simulink model "actuator_sensor"  (R2017a)
settings: Solver=ode45  StartTime=0.0  StopTime=150  FixedStep=1e-4  RelTol=1e-6  EnableMultiTasking=on
values from neighbouring files (symbols this model uses):
  A = [3.7451e-15 7.6548e-6 0 0;-4.0887e-6 -6.5527e-2 0 0;     2.3773e-6 5.9026e-4 -0.1426 0;-8.1593e-14 -5.5355e-2 18.216 0.08333];eig(A)    [boiler.m]    (also in boiler2.m = [3.7451e-15 7.6548e-6 0 0;-4.0887e-6 -6.5527e-2 0 0;     2.3)
  A0 = [zeros(3,2);A0]    [boiler2.m]
  A_m = [-0.01 0 0;0 -0.02 0;0 0 -0.03]    [boiler.m]    (also in boiler2.m)
  Ab = [A zeros(n,psi_s);Omega*C_f -Omega]    [boiler2.m]
  alpha_0 = 8.0314    [boiler.m]    (also in boiler2.m)
  alpha_1 = 1.4713    [boiler.m]    (also in boiler2.m)
  B = [0.0015 -0.0015 -6.9678e-12;-5.9548e-5 -9.0316e-5 5.9647e-11;     3.4622e-5 5.2512e-5 3.2492e-11;-0.0167 0.0239 -1.0733e-9]    [boiler.m]    (also in boiler2.m)
  B_m = [1 0 0 ; 0 1 0 ; 0 0 1]    [boiler.m]    (also in boiler2.m)
  Bb = [B;zeros(psi_s,m)]    [boiler2.m]
  Bound = 1e-3    (= 0.001)    [boiler.m]    (also in boiler2.m)
  C = [0.05 -0.0484 6.7129 0.05;0 1 0 0]    [boiler.m]    (also in boiler2.m)
  C_m = [0 1 0;1 0 0]    [boiler.m]    (also in boiler2.m)
  Cb = [C_h zeros(p-psi_s,psi_s);zeros(psi_s,n) eye(psi_s)]    [boiler2.m]
  D = [0 0 0 ; 0 0 0]    [boiler.m]    (also in boiler2.m = [0 0 0 20]')
  Db_p = T*Db    [boiler2.m]
  E = dB    [boiler2.m]
  f_a = 10    [boiler2.m]
  f_s = 0.1    [boiler2.m]
  FTC_factor = 1    [boiler2.m]
  G = [0.968,-114.258,-1;1,0,0;0,1,0;0,0,1]    [boiler.m]    (also in boiler2.m)
  gamma = 0.0013    [boiler.m]    (also in boiler2.m)
  Gamma = 1*diag([1,1,1])    [boiler.m]    (also in boiler2.m)
  H = [-0.00264411452837401,0.276368234354978,0.00485669922298695;-0.00212093673792562,0.126828183853013,0.00297639139790861;-11263.6759461726,221638.898137783,1282.33499200163]    [boiler.m]    (also in boiler2.m)
  k = norm(D2)*pa + eta1    [boiler2.m]
  K_D = [0.0691 0 0 0.0691;0 0.0691 0 0;0 0 0.0691 0]    [boiler.m]    (also in boiler2.m)
  K_I = 2*[eye(3),[1;0;0]]    [boiler.m]    (also in boiler2.m)
  K_P = .1*[eye(3),[1;0;0]]    [boiler.m]    (also in boiler2.m)
  K_S = 0.01*eye(3)    [boiler.m]    (also in boiler2.m)
  M = [0.322180266848393,-23.9048793908242,-0.198387888997022;0.273413353570640,-16.9472760226837,-0.136907357417107;1077571.96327408,-5503793.87571974,-55561.6496148715]    [boiler.m]    (also in boiler2.m)
  N = [0 1]'    [boiler2.m]
  Omega = 10    [boiler2.m]
  P0 = eye(p)    [boiler2.m]
  sai = 1e-3    (= 0.001)    [boiler2.m]
  T = [[eye(3) zeros(3,2)];Cb]    [boiler2.m]
  um_factor = 1    [boiler.m]    (also in boiler2.m = 0)
settings Model: Creator=Mohmmad Mousavi  LastModifiedBy=Mohmmad Mousavi
settings DataIOCC: LimitDataPoints=on  SaveFormat=Array
settings OptimizationCC: LifeSpan=inf
settings DebuggingCC: SFUnexpectedBacktrackingDiag=warning  SFNoUnconditionalDefaultTransitionDiag=warning  SFExecutionAtInitializationDiag=none
settings HardwareCC: ProdBitPerPointer=32  ProdBitPerSizeT=32  ProdBitPerPtrDiffT=32  ProdLargestAtomicFloat=None  ProdIntDivRoundTo=Undefined  ProdEndianess=Unspecified  ProdWordSize=32  ProdHWDeviceType=32-bit Generic
settings ModelReferenceCC: PropagateSignalLabelsOutOfModel=off
settings GRTTargetCC: TargetLangStandard=C89/C90 (ANSI)  GeneratePreprocessorConditionals=Disable all
settings ConfigComp: CovMetricSettings=dw  CovHtmlReporting=on  CovSaveCumulativeToWorkspaceVar=on  CovSaveSingleToWorkspaceVar=on  CovExternalEMLEnable=off

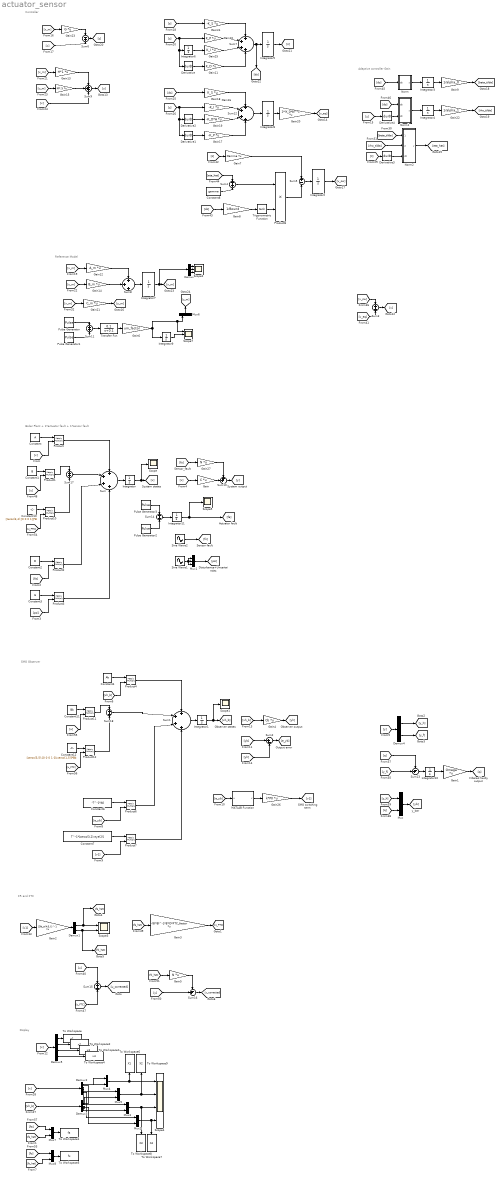
== system actuator_sensor ==
  note: FR and FTC
  note: Display
  note: Boiler Plant + 1*actuator fault + 1*sensor fault
  note: SMO Observer
  note: Controller
  note: Adaptive controller Gain
  note: Reference Model
  Constant : Constant  Value=A
  Constant1 : Constant  Value=B
  Constant10 : Constant  Value=[zeros(3,4);[0 0 0 1]]*B
  Constant11 : Constant  Value=Bb
  Constant12 : Constant  Value=[zeros(3,5);[0 0 0 1 0];zeros(1,5)]*Bb
  Constant2 : Constant  Value=D
  Constant3 : Constant  Value=E
  Constant4 : Constant  Value=Ab
  Constant6 : Constant  Value=-T^-1*A0
  Constant7 : Constant  Value=T^-1*[zeros(3,2);eye(2)]
  Constant8 : Constant  Value=gamma
  Demux : Demux  Outputs=3
  Demux1 : Demux  Outputs=2
  Demux2 : Demux  Outputs=n
  Demux3 : Demux  Outputs=5
  Demux4 : Demux  Outputs=2
  Demux5 : Demux  Outputs=n
  Derivative{,1..4} (5 alike) : Derivative
  Gain : Gain  Gain=C  Multiplication=Matrix(K*u)
  Gain1 : Gain  Gain=Omega  Multiplication=Matrix(K*u)
  Gain10 : Gain  Gain=K_P  Multiplication=Matrix(K*u)
  Gain11 : Gain  Gain=K_D  Multiplication=Matrix(K*u)
  Gain12 : Gain  Gain=A_m  Multiplication=Matrix(K*u)
  Gain13 : Gain  Gain=H*1  Multiplication=Matrix(K*u)
  Gain14 : Gain  Gain=B_m  Multiplication=Matrix(K*u)
  Gain15 : Gain  Gain=M*.5  Multiplication=Matrix(K*u)
  Gain16 : Gain  Gain=-K_I  Multiplication=Matrix(K*u)
  Gain17 : Gain  Gain=-K_P  Multiplication=Matrix(K*u)
  Gain18 : Gain  Gain=K_S  Multiplication=Matrix(K*u)
  Gain19 : Gain  Gain=-K_D*A  Multiplication=Matrix(K*u)
  Gain2 : Gain  Gain=[Db_p(4:5,:)]^-1  Multiplication=Matrix(K*u)
  Gain20 : Gain  Gain=2*(K_D*B)^-1  Multiplication=Matrix(K*u)
  Gain21 : Gain  Gain=C_m  Multiplication=Matrix(K*u)
  Gain22 : Gain  Gain=1/alpha_1
  Gain23 : Gain  Gain=G  Multiplication=Matrix(K*u)
  Gain24 : Gain  Gain=-K_S  Multiplication=Matrix(K*u)
  Gain25 : Gain  Gain=K_I  Multiplication=Matrix(K*u)
  Gain26 : Gain  Gain=k*P0  Multiplication=Matrix(K*u)
  Gain27 : Gain  Gain=N  Multiplication=Matrix(K*u)
  Gain3 : Gain  Gain=-(B'*B)^-1*B'*D*FTC_factor  Multiplication=Matrix(K*u)
  Gain4 : Gain  Gain=Cb  Multiplication=Matrix(K*u)
  Gain5 : Gain  Gain=N  Multiplication=Matrix(K*u)
  Gain6 : Gain  Gain=um_factor
  Gain7 : Gain  Gain=Gamma  Multiplication=Matrix(K*u)
  Gain8 : Gain  Gain=1/Bound
  Gain9 : Gain  Gain=1/alpha_0
  Integrator : Integrator  InitialCondition=[25 30 9 -950]*0.5
  Integrator1 : Integrator  InitialCondition=[25 30*.5 9*0.5 -950 0]*0.5
  Integrator{3..6,8,10..11} (7 alike) : Integrator
  Integrator2 : Integrator  InitialCondition=zeros(3,1)
  Integrator7 : Integrator  InitialCondition=[ 60 9 0.05]
  Integrator9 : Integrator  InitialCondition=35
  MATLAB Function : MATLAB Function  TreatAsAtomicUnit=on
  Mux{,2..5,7..8} (7 alike) : Mux  Inputs=2
  Mux1 : Mux  Inputs=3
  Mux6 : Mux  Inputs=3
  Norm : MATLAB Function  TreatAsAtomicUnit=on
  Norm1 : MATLAB Function  TreatAsAtomicUnit=on
  Norm2 : MATLAB Function  TreatAsAtomicUnit=on
  Product{,1..4,6..7,10..12} (10 alike) : Product  Multiplication=Matrix(*)
  Product8 : Product
  Pulse Generator : DiscretePulseGenerator  PulseType=Time based  Amplitude=1.9  Period=100  PulseWidth=50
  Pulse Generator1 : DiscretePulseGenerator  PulseType=Time based  Amplitude=-.5  Period=100  PulseWidth=50  PhaseDelay=50
  Pulse Generator2 : DiscretePulseGenerator  PulseType=Time based  Amplitude=-f_a/5  Period=10  PulseWidth=50  PhaseDelay=5
  Pulse Generator3 : DiscretePulseGenerator  PulseType=Time based  Amplitude=f_a/5  Period=10  PulseWidth=50
  Scope : Scope
  Scope1 : Scope
  Scope2 : Scope  NumInputPorts=3
  Scope3 : Scope  NumInputPorts=2
  Scope4 : Scope  NumInputPorts=4
  Scope5 : Scope
  Scope7 : Scope  NumInputPorts=3
  Sine Wave1 : Sin  Amplitude=sai  SampleTime=0
  Sine Wave2 : Sin  Amplitude=f_s  SampleTime=0
  Sum{,1,7,12} (4 alike) : Sum  Inputs=++++
  Sum10 : Sum  Inputs=++|
  Sum{3..4,11,14..15,17..18} (7 alike) : Sum
  Sum13 : Sum  Inputs=-+|
  Sum16 : Sum  Inputs=-+|
  Sum2 : Sum  Inputs=|+-
  Sum5 : Sum  Inputs=+-
  Sum6 : Sum  Inputs=-+
  Sum8 : Sum  Inputs=+++
  Sum9 : Sum  Inputs=+++
  To Workspace : ToWorkspace  VariableName=x1  SaveFormat=Timeseries  SampleTime=-1
  To Workspace1 : ToWorkspace  VariableName=fa  SaveFormat=Timeseries  SampleTime=-1
  To Workspace2 : ToWorkspace  VariableName=x2  SaveFormat=Timeseries  SampleTime=-1
  To Workspace3 : ToWorkspace  VariableName=x3  SaveFormat=Timeseries  SampleTime=-1
  To Workspace4 : ToWorkspace  VariableName=x4  SaveFormat=Timeseries  SampleTime=-1
  To Workspace5 : ToWorkspace  VariableName=fs  SaveFormat=Timeseries  SampleTime=-1
  To Workspace6 : ToWorkspace  VariableName=X1  SaveFormat=Timeseries  SampleTime=-1
  To Workspace7 : ToWorkspace  VariableName=X4  SaveFormat=Timeseries  SampleTime=-1
  To Workspace8 : ToWorkspace  VariableName=X3  SaveFormat=Timeseries  SampleTime=-1
  To Workspace9 : ToWorkspace  VariableName=X2  SaveFormat=Timeseries  SampleTime=-1
  Transfer Fcn : TransferFcn  Numerator=[0.1]  Denominator=[1 0.1]
  Trigonometric Function : Trigonometry  Operator=tanh
  wires:
  Constant/1 -> Product/1
  [x] -> Product/2
  Product/1 -> Sum/1
  Constant1/1 -> Product1/1
  [u] -> Product1/2
  Constant2/1 -> Product2/1
  [fa] -> Product2/2
  Product2/1 -> Sum/3
  Constant3/1 -> Product3/1
  [psi] -> Product3/2
  Sum/1 -> Integrator/1
  Integrator/1 -> Scope/1, [x]
  [x] -> Gain/1
  Constant4/1 -> Product4/1
  [xh_b] -> Product4/2
  Product4/1 -> Sum1/1
  Constant6/1 -> Product6/1
  [e_yb] -> Product6/2
  Product6/1 -> Sum1/3
  Constant7/1 -> Product7/1
  [v1] -> Product7/2
  Product7/1 -> Sum1/4
  Sum1/1 -> Integrator1/1
  Integrator1/1 -> Scope1/1, [xh_b]
  Sum2/1 -> [e_yb]
  [yb] -> Sum2/1
  Gain4/1 -> [yh]
  [xh_b] -> Gain4/1
  [yh] -> Sum2/2
  [e_yb] -> MATLAB Function/1(u)
  MATLAB Function/1(v) -> Gain26/1
  [x] -> Demux2/1
  [xh_b] -> Demux3/1
  Mux2/1 -> To Workspace7/1, Scope4/4
  Mux3/1 -> Scope4/3, To Workspace8/1
  Mux5/1 -> To Workspace9/1, Scope4/2
  Mux4/1 -> To Workspace6/1, Scope4/1
  Demux2/1 -> Mux4/1
  Demux3/1 -> Mux4/2
  Demux2/2 -> Mux5/1
  Demux3/2 -> Mux5/2
  Demux2/3 -> Mux3/1
  Demux3/3 -> Mux3/2
  Demux2/4 -> Mux2/1
  Demux3/4 -> Mux2/2
  Sum3/1 -> [v]
  [v_sw] -> Sum3/1
  [v_eq] -> Sum3/2
  [s] -> Gain7/1
  Gain7/1 -> Sum5/1
  Integrator2/1 -> [v_sw]
  [ds] -> Gain8/1
  Constant8/1 -> Sum4/2
  Gain8/1 -> Trigonometric Function/1
  Sum4/1 -> Product8/1
  Trigonometric Function/1 -> Product8/2
  Product8/1 -> Sum5/2
  Sum5/1 -> Integrator2/1
  Integrator3/1 -> Gain9/1
  Gain9/1 -> [beta_tilda]
  [ds] -> Norm/1(ds)
  Norm/1(y) -> Integrator3/1
  Integrator4/1 -> Gain22/1
  Gain22/1 -> [rho_tilda]
  [ds] -> Norm1/1(ds)
  Norm1/1(y) -> Integrator4/1
  Sum6/1 -> [z]
  [x] -> Sum6/2
  [x_m] -> Gain23/1
  Gain23/1 -> Sum6/1
  [s] -> Gain24/1
  Integrator6/1 -> Gain25/1
  Gain10/1 -> Sum7/2
  Gain24/1 -> Sum7/1
  Gain25/1 -> Sum7/3
  Sum7/1 -> Integrator5/1, [ds]
  Integrator5/1 -> [s]
  [z] -> Derivative/1, Integrator6/1, Gain10/1
  Derivative/1 -> Gain11/1
  Gain11/1 -> Sum7/4
  [x_m] -> Gain12/1
  [u_m] -> Gain14/1
  Gain14/1 -> Sum8/2
  Gain12/1 -> Sum8/1
  Sum8/1 -> Integrator7/1
  Integrator7/1 -> Demux/1, [x_m]
  Mux6/1 -> [u_m]
  [x_m] -> Gain13/1
  [u_m] -> Gain15/1
  Gain13/1 -> Sum9/1
  Gain15/1 -> Sum9/2
  [v] -> Sum9/3
  Sum9/1 -> [u]
  Demux/1 -> Scope2/1
  Demux/2 -> Scope2/2
  Demux/3 -> Scope2/3
  [ds] -> Gain18/1
  Derivative2/1 -> Gain19/1
  Gain16/1 -> Sum12/2
  Gain18/1 -> Sum12/1
  Sum12/1 -> Integrator8/1
  [z] -> Derivative2/1, Derivative1/1, Gain16/1
  Derivative1/1 -> Gain17/1
  Gain17/1 -> Sum12/4
  Integrator8/1 -> Gain20/1
  Gain20/1 -> [v_eq]
  Norm2/1(y) -> [eta_hat]
  [beta_tilda] -> Norm2/1(beta_tilda)
  [z] -> Derivative3/1
  Derivative3/1 -> Norm2/3(dz)
  [z] -> Derivative4/1
  Derivative4/1 -> Norm1/2(dz)
  [x_m] -> Gain21/1
  Gain21/1 -> [y_m]
  Pulse Generator/1 -> Sum11/1
  Gain19/1 -> Sum12/3
  Integrator9/1 -> Scope7/2
  Pulse Generator1/1 -> Sum11/2
  Gain6/1 -> Integrator9/1, Scope7/1, Mux6/1
  [eta_hat] -> Sum4/1
  [rho_tilda] -> Norm2/2(rho_tilda)
  Sum11/1 -> Transfer Fcn/1
  Transfer Fcn/1 -> Gain6/1
  Gain26/1 -> [v1]
  Integrator11/1 -> [fa], Scope5/1
  Sine Wave2/1 -> [fs]
  Sum10/1 -> [y]
  Gain/1 -> Sum10/2
  [fs] -> Gain27/1
  Gain27/1 -> Sum10/1
  [y] -> Demux4/1
  Demux4/1 -> [y_h]
  Demux4/2 -> [y_f]
  Sum13/1 -> Integrator10/1
  [y_f] -> Sum13/2
  Integrator10/1 -> Gain1/1
  Gain1/1 -> [q]
  [q] -> Sum13/1
  [y_h] -> Mux/1
  [q] -> Mux/2
  Mux/1 -> [yb]
  Sum14/1 -> Integrator11/1
  Pulse Generator3/1 -> Sum14/1
  Pulse Generator2/1 -> Sum14/2
  Mux1/1 -> [psi]
  Sine Wave1/1 -> Mux1/3, Mux1/1, Mux1/2
  Product3/1 -> Sum/4
  [x] -> Demux5/1
  Demux5/1 -> To Workspace/1
  Demux5/2 -> To Workspace2/1
  Demux5/3 -> To Workspace3/1
  Demux5/4 -> To Workspace4/1
  Sum15/1 -> [u_corrected]
  [u] -> Sum15/1
  [u_FTC] -> Sum15/2
  Gain3/1 -> [u_FTC]
  Demux1/1 -> [fa_hat], Scope3/1
  Gain2/1 -> Demux1/1
  Demux1/2 -> [fs_hat], Scope3/2
  [v1] -> Gain2/1
  [fa_hat] -> Gain3/1
  [fs_hat] -> Gain5/1
  Gain5/1 -> Sum16/1
  [y] -> Sum16/2
  Sum16/1 -> [y_corrected]
  Product1/1 -> Sum17/1
  Constant10/1 -> Product10/1
  [u_FTC] -> Product10/2
  Product10/1 -> Sum17/2
  Sum17/1 -> Sum/2
  Constant11/1 -> Product11/1
  [u] -> Product11/2
  Product11/1 -> Sum18/1
  Constant12/1 -> Product12/1
  [u_FTC] -> Product12/2
  Product12/1 -> Sum18/2
  Sum18/1 -> Sum1/2
  [fa] -> Mux7/1
  [fa_hat] -> Mux7/2
  [fs] -> Mux8/1
  [fs_hat] -> Mux8/2
  Mux8/1 -> To Workspace5/1
  Mux7/1 -> To Workspace1/1

== matlab function actuator_sensor/Norm ==
  data: ds input; y output
function y = fcn(ds)
%#codegen

y = norm(ds);

== matlab function actuator_sensor/MATLAB Function ==
  data: u input; v output
function v = fcn(u)
%#codegen
delta = 1e-2;
v = [0;0];
v(1) = u(1)/(abs(u(1))+delta);
v(2) = u(2)/(abs(u(2))+delta);

== matlab function actuator_sensor/Norm1 ==
  data: ds input; y output; dz input
function y = fcn(ds,dz)
%#codegen

y = norm(ds)*norm(dz);

== matlab function actuator_sensor/Norm2 ==
  data: beta_tilda input; y output; rho_tilda input; dz input
function y = fcn(beta_tilda,rho_tilda,dz)
%#codegen

y = 0*(beta_tilda + rho_tilda*norm(dz));
